simulink model "Punto1_2"  (R2022b)
settings: Solver=VariableStepAuto  StartTime=0.0  StopTime=10.0  RelTol=1e-3
settings Model: Creator=prestamour  LastModifiedBy=laura

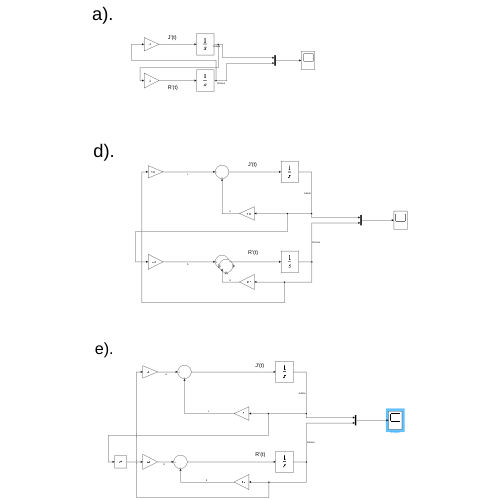
[thumbnail: Simulink's stored preview of the top-level diagram]
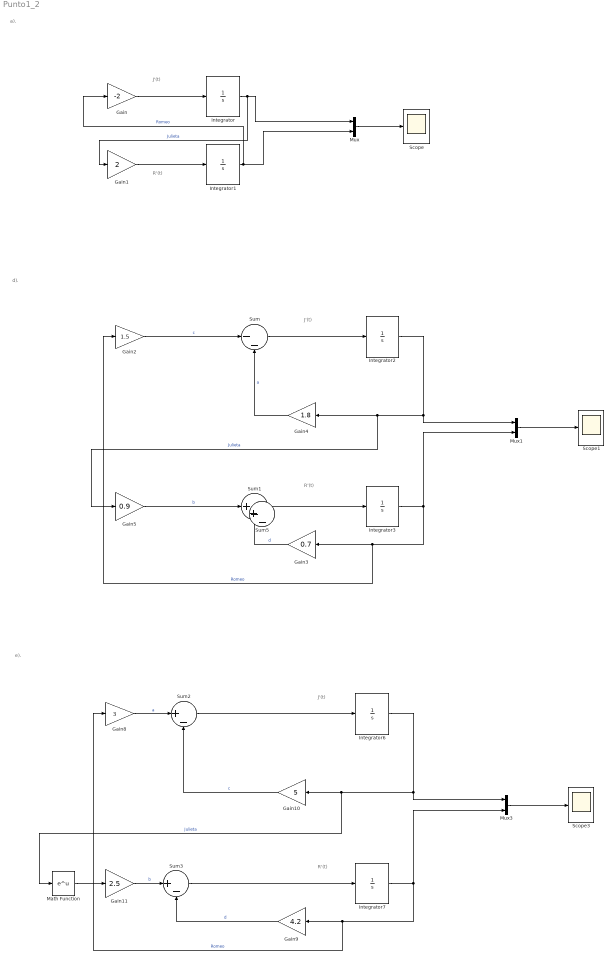
== system Punto1_2 ==
  note: e).
  note: a).
  note: R'(t)
  note: J'(t)
  note: J'(t)
  note: R'(t)
  note: d).
  note: R'(t)
  note: J'(t)
  Gain : Gain  Gain=-2
  Gain1 : Gain  Gain=2
  Gain10 : Gain  Gain=5
  Gain11 : Gain  Gain=2.5
  Gain2 : Gain  Gain=1.5
  Gain3 : Gain  Gain=0.7
  Gain4 : Gain  Gain=1.8
  Gain5 : Gain  Gain=0.9
  Gain8 : Gain  Gain=3
  Gain9 : Gain  Gain=4.2
  Integrator{,1,3,7} (4 alike) : Integrator
  Integrator2 : Integrator  InitialCondition=1
  Integrator6 : Integrator  InitialCondition=1
  Math Function : Math
  Mux : Mux  Inputs=2
  Mux1 : Mux  Inputs=2
  Mux3 : Mux  Inputs=2
  Scope : Scope
  Scope1 : Scope
  Scope3 : Scope
  Sum : Sum  Inputs=|--
  Sum{1..3,5} (4 alike) : Sum  Inputs=|+-
  wires:
  Gain1/1 -> Integrator1/1
  Gain/1 -> Integrator/1
  Integrator/1 -> Mux/1, Gain1/1  "Julieta"
  Integrator1/1 -> Gain/1, Mux/2  "Romeo"
  Mux/1 -> Scope/1
  Mux1/1 -> Scope1/1
  Gain2/1 -> Sum/1  "c"
  Sum/1 -> Integrator2/1
  Gain4/1 -> Sum/2  "a"
  Gain3/1 -> Sum1/2  "d"
  Gain5/1 -> Sum1/1  "b"
  Integrator2/1 -> Mux1/1, Gain5/1, Gain4/1  "Julieta"
  Integrator3/1 -> Mux1/2, Gain2/1, Gain3/1  "Romeo"
  Sum1/1 -> Integrator3/1
  Mux3/1 -> Scope3/1
  Gain10/1 -> Sum2/2  "c"
  Sum3/1 -> Integrator7/1
  Integrator7/1 -> Mux3/2, Gain8/1, Gain9/1  "Romeo"
  Gain9/1 -> Sum3/2  "d"
  Integrator6/1 -> Mux3/1, Math Function/1, Gain10/1  "Julieta"
  Gain8/1 -> Sum2/1  "a"
  Gain11/1 -> Sum3/1  "b"
  Sum2/1 -> Integrator6/1
  Math Function/1 -> Gain11/1
